simulink model "Zhang2004QP"  (Simulink 8.6)
settings: Solver=FixedStepAuto  StartTime=0.0  StopTime=20  FixedStep=Ts  RelTol=1e-3
InitFcn:
  | Zhang2004QP_init;
undefined symbols (not defined in the file or in its folder): CONFIG, DiscIntNeverNeededParam, model, ROBOT_DOF, Ts
libraries: WBToolboxLibrary x14
settings Model: Creator=marie  LastModifiedBy=marie
settings DataIOCC: SaveFormat=Dataset  SignalLoggingSaveFormat=Dataset
settings OptimizationCC: ExpressionDepthLimit=128
settings DebuggingCC: UnderspecifiedInitializationDetection=Simplified  MergeDetectMultiDrivingBlocksExec=error  SolverPrmCheckMsg=none  FcnCallInpInsideContextMsg=EnableAllAsError  StateNameClashWarn=none
settings HardwareCC: ProdBitPerPointer=64  ProdLargestAtomicFloat=Float  ProdIntDivRoundTo=Zero  ProdEndianess=LittleEndian  ProdWordSize=64  ProdHWDeviceType=Intel->x86-64 (Windows64)
settings GRTTargetCC: GeneratePreprocessorConditionals=Use local settings  CombineOutputUpdateFcns=on  GRTInterface=off
settings ConfigComp: CovModelRefEnable=off

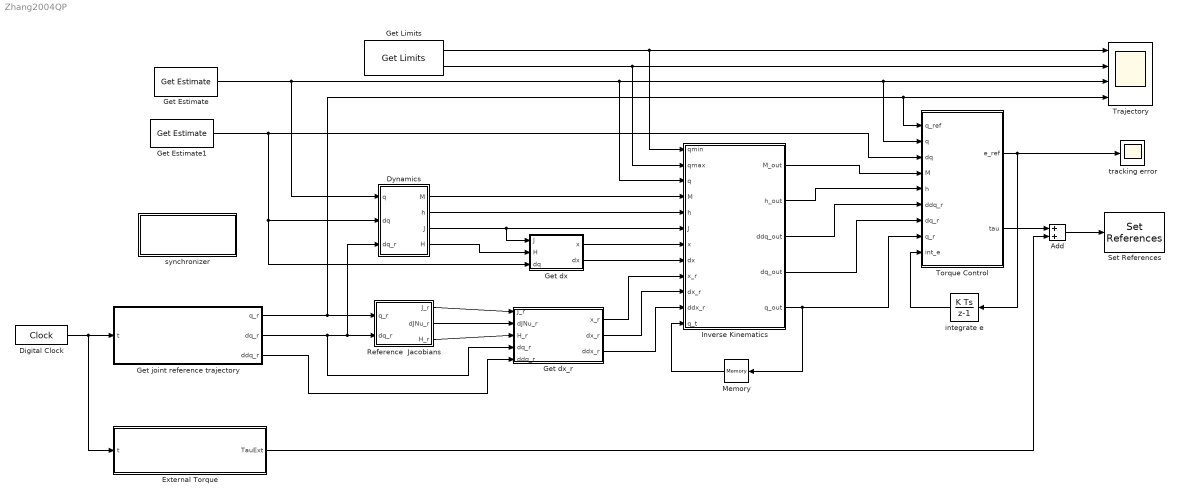
== system Zhang2004QP ==
  Add : Sum
  Digital Clock : DigitalClock  SampleTime=Ts
  Dynamics : Subsystem
  External Torque : MATLAB Function  TreatAsAtomicUnit=on
  Get Estimate : WBToolboxLibrary/wholeBodyStates/Get Estimate  estimateType=Joints Position  robotName=WBT_robotName  localName=WBT_modelName  wbiFile=WBT_wbiFilename  wbiList=WBT_wbiList
  Get Estimate1 : WBToolboxLibrary/wholeBodyStates/Get Estimate  estimateType=Joints Velocity  robotName=WBT_robotName  localName=WBT_modelName  wbiFile=WBT_wbiFilename  wbiList=WBT_wbiList
  Get Limits : WBToolboxLibrary/wholeBodyStates/Get Limits  limitsType=Position  robotName=WBT_robotName  localName=WBT_modelName  wbiFile=WBT_wbiFilename  wbiList=WBT_wbiList
  Get dx : MATLAB Function  TreatAsAtomicUnit=on
  Get dx_r : MATLAB Function  TreatAsAtomicUnit=on
  Get joint reference trajectory : MATLAB Function  TreatAsAtomicUnit=on
  Inverse Kinematics : MATLAB Function  TreatAsAtomicUnit=on
  Memory : Memory  InheritSampleTime=on
  Reference  Jacobians : Subsystem
  Set References : WBToolboxLibrary/wholeBodyActuators/Set References  controlType=Torque  robotName=WBT_robotName  localName=WBT_modelName  wbiFile=WBT_wbiFilename  wbiList=WBT_wbiList
  Torque Control : MATLAB Function  TreatAsAtomicUnit=on
  Trajectory : Scope  NumInputPorts=4
  integrate e : DiscreteIntegrator  InitialConditionSetting=State (most efficient)  SampleTime=Ts  ICPrevOutput=DiscIntNeverNeededParam  ICPrevScaledInput=DiscIntNeverNeededParam
  synchronizer : Subsystem
      mask Display: disp('SYNCHRONIZER')
  tracking error : Scope
  wires:
  Digital Clock/1 -> External Torque/1(t), Get joint reference trajectory/1(t)
  Torque Control/1(e_ref) -> integrate e/1, tracking error/1
  integrate e/1 -> Torque Control/9(int_e)
  Get Estimate/1 -> Dynamics/1(q), Trajectory/3, Torque Control/2(q), Inverse Kinematics/3(q)
  Get Estimate1/1 -> Get dx/3(dq), Dynamics/2(dq), Torque Control/3(dq)
  Get joint reference trajectory/1(q_r) -> Reference  Jacobians/1(q_r), Trajectory/4, Torque Control/1(q_ref)
  Get joint reference trajectory/2(dq_r) -> Reference  Jacobians/2(dq_r), Dynamics/3(dq_r), Get dx_r/4(dq_r)
  Get joint reference trajectory/3(ddq_r) -> Get dx_r/5(ddq_r)
  Get Limits/1 -> Trajectory/1, Inverse Kinematics/1(qmin)
  Get Limits/2 -> Trajectory/2, Inverse Kinematics/2(qmax)
  Dynamics/1(M) -> Inverse Kinematics/4(M)
  Dynamics/2(h) -> Inverse Kinematics/5(h)
  Reference  Jacobians/1(J_r) -> Get dx_r/1(J_r)
  Reference  Jacobians/2(dJNu_r) -> Get dx_r/2(dJNu_r)
  Dynamics/3(J) -> Inverse Kinematics/6(J), Get dx/1(J)
  Reference  Jacobians/3(H_r) -> Get dx_r/3(H_r)
  Dynamics/4(H) -> Get dx/2(H)
  Get dx_r/1(x_r) -> Inverse Kinematics/9(x_r)
  Get dx_r/2(dx_r) -> Inverse Kinematics/10(dx_r)
  Get dx_r/3(ddx_r) -> Inverse Kinematics/11(ddx_r)
  Get dx/1(x) -> Inverse Kinematics/7(x)
  Get dx/2(dx) -> Inverse Kinematics/8(dx)
  Inverse Kinematics/3(ddq_out) -> Torque Control/6(ddq_r)
  Inverse Kinematics/5(q_out) -> Torque Control/8(q_r), Memory/1
  Memory/1 -> Inverse Kinematics/12(q_t)
  Inverse Kinematics/1(M_out) -> Torque Control/4(M)
  Inverse Kinematics/2(h_out) -> Torque Control/5(h)
  Inverse Kinematics/4(dq_out) -> Torque Control/7(dq_r)
  Torque Control/2(tau) -> Add/1
  External Torque/1(TauExt) -> Add/2
  Add/1 -> Set References/1

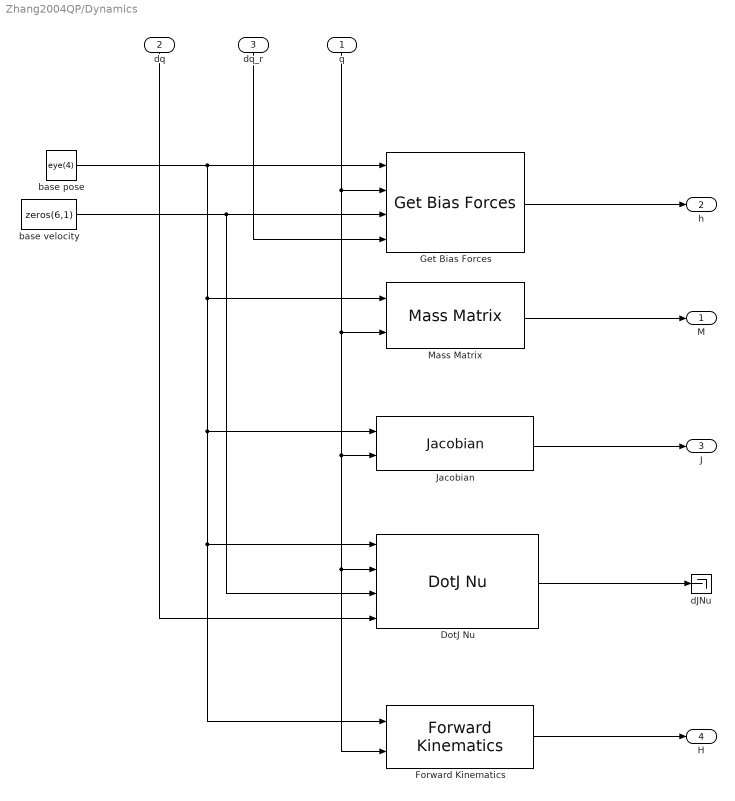
== system Zhang2004QP/Dynamics ==
  q : Inport
  dq : Inport  Port=2
  dq_r : Inport  Port=3
  DotJ Nu : WBToolboxLibrary/wholeBodyModel/Jacobians/DotJ Nu  frameName='r_sole'  robotName=WBT_robotName  localName=WBT_modelName  wbiFile=WBT_wbiFilename  wbiList=WBT_wbiList
  Forward Kinematics : WBToolboxLibrary/wholeBodyModel/Kinematics/Forward Kinematics  frameName='r_sole'  robotName=WBT_robotName  localName=WBT_modelName  wbiFile=WBT_wbiFilename  wbiList=WBT_wbiList
  Get Bias Forces : WBToolboxLibrary/wholeBodyModel/Dynamics/Get Bias Forces  robotName=WBT_robotName  localName=WBT_modelName  wbiFile=WBT_wbiFilename  wbiList=WBT_wbiList
  Jacobian : WBToolboxLibrary/wholeBodyModel/Jacobians/Jacobian  frameName='r_sole'  robotName=WBT_robotName  localName=WBT_modelName  wbiFile=WBT_wbiFilename  wbiList=WBT_wbiList
  Mass Matrix : WBToolboxLibrary/wholeBodyModel/Dynamics/Mass Matrix  robotName=WBT_robotName  localName=WBT_modelName  wbiFile=WBT_wbiFilename  wbiList=WBT_wbiList
  base pose : Constant  Value=eye(4)
  base velocity : Constant  Value=zeros(6,1)
  dJNu : Terminator
  M : Outport
  h : Outport  Port=2
  J : Outport  Port=3
  H : Outport  Port=4
  wires:
  base pose/1 -> Get Bias Forces/1, Forward Kinematics/1, DotJ Nu/1, Jacobian/1, Mass Matrix/1
  dq_r/1 -> Get Bias Forces/4
  Mass Matrix/1 -> M/1
  base velocity/1 -> DotJ Nu/3, Get Bias Forces/3
  Get Bias Forces/1 -> h/1
  q/1 -> DotJ Nu/2, Forward Kinematics/2, Jacobian/2, Mass Matrix/2, Get Bias Forces/2
  dq/1 -> DotJ Nu/4
  Jacobian/1 -> J/1
  DotJ Nu/1 -> dJNu/1
  Forward Kinematics/1 -> H/1

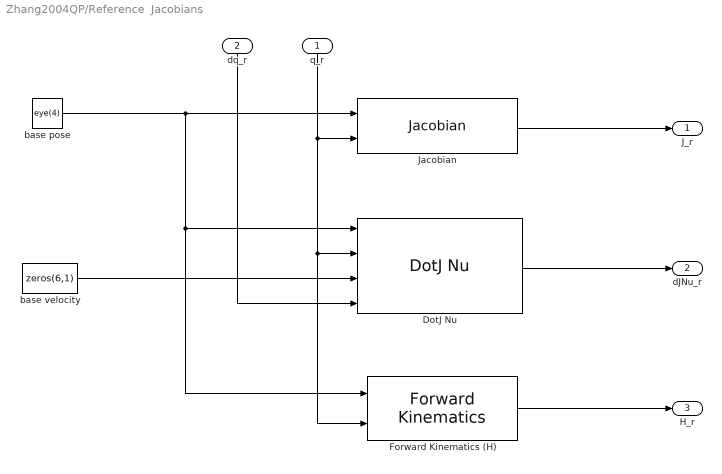
== system Zhang2004QP/Reference  Jacobians ==
  q_r : Inport
  dq_r : Inport  Port=2
  DotJ Nu : WBToolboxLibrary/wholeBodyModel/Jacobians/DotJ Nu  frameName='r_sole'  robotName=WBT_robotName  localName=WBT_modelName  wbiFile=WBT_wbiFilename  wbiList=WBT_wbiList
  Forward Kinematics (H) : WBToolboxLibrary/wholeBodyModel/Kinematics/Forward Kinematics  frameName='r_sole'  robotName=WBT_robotName  localName=WBT_modelName  wbiFile=WBT_wbiFilename  wbiList=WBT_wbiList
  Jacobian : WBToolboxLibrary/wholeBodyModel/Jacobians/Jacobian  frameName='r_sole'  robotName=WBT_robotName  localName=WBT_modelName  wbiFile=WBT_wbiFilename  wbiList=WBT_wbiList
  base pose : Constant  Value=eye(4)
  base velocity : Constant  Value=zeros(6,1)
  J_r : Outport
  dJNu_r : Outport  Port=2
  H_r : Outport  Port=3
  wires:
  DotJ Nu/1 -> dJNu_r/1
  Jacobian/1 -> J_r/1
  q_r/1 -> Jacobian/2, DotJ Nu/2, Forward Kinematics (H)/2
  base velocity/1 -> DotJ Nu/3
  base pose/1 -> Jacobian/1, Forward Kinematics (H)/1, DotJ Nu/1
  dq_r/1 -> DotJ Nu/4
  Forward Kinematics (H)/1 -> H_r/1

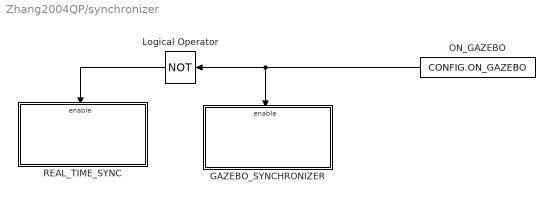
== system Zhang2004QP/synchronizer ==
  GAZEBO_SYNCHRONIZER : Subsystem
  Logical Operator : Logic  Operator=NOT  AllPortsSameDT=off  OutDataTypeStr=boolean
  "ON_GAZEBO " : Constant  Value=CONFIG.ON_GAZEBO
  REAL_TIME_SYNC : Subsystem
  wires:
  Logical Operator/1 -> REAL_TIME_SYNC/Enable
  "ON_GAZEBO "/1 -> GAZEBO_SYNCHRONIZER/Enable, Logical Operator/1

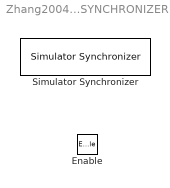
== system Zhang2004QP/synchronizer/GAZEBO_SYNCHRONIZER ==
  Enable : EnablePort
  Simulator Synchronizer : WBToolboxLibrary/Utilities/Simulator Synchronizer  period=CONFIG.Ts  serverPortName='/clock/rpc'  clientPortName='/WBT_synchronizer/rpc:o'

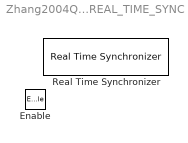
== system Zhang2004QP/synchronizer/REAL_TIME_SYNC ==
  Enable : EnablePort
  Real Time Synchronizer : WBToolboxLibrary/Utilities/Real Time Synchronizer  period=CONFIG.Ts

== matlab function Torque Control ==
  data: e_ref output double; q_ref input double; q input double; dq input double; M input double; h input double; ddq_r input double; dq_r input double; q_r input double; tau output double; int_e input double; ROBOT_DOF parameter double; model parameter double
function [e_ref, tau] = jointEvolutionControlFCN(q_ref, q, dq, M, h, ddq_r, dq_r, q_r, int_e, ROBOT_DOF, model)


[tau, e_ref] = jointEvolutionControl(q_ref, q, dq, M, h, ddq_r, dq_r, q_r, int_e, ROBOT_DOF, model);

== matlab function Get joint reference trajectory ==
  data: q_r output double; dq_r output double; ddq_r output double; t input double; model parameter double
function [q_r, dq_r, ddq_r] = generateReferenceTrajectoriesFCN(t, model)

[q_r, dq_r, ddq_r]  = generateReferenceTrajectories(t, model);

== matlab function Get dx_r ==
  data: x_r output double; J_r input double; dx_r output double; dJNu_r input double; H_r input double; dq_r input double; ddq_r input double; ddx_r output double
function [x_r, dx_r, ddx_r] = get_dx_rFCN(J_r, dJNu_r, H_r, dq_r, ddq_r)

%base velocity and acceleration = 0
Nu_r = [zeros(6,1); dq_r];
dNu_r = [zeros(6,1); ddq_r];

[x_r, dx_r, ddx_r] = get_dx(J_r, dJNu_r, H_r, Nu_r, dNu_r);

end

== matlab function Inverse Kinematics ==
  data: qmin input double; qmax input double; q input double; M input double; h input double; J input double; x input double; dx input double; x_r input double; M_out output double; h_out output double; ddq_out output double; dq_out output double; q_out output double; dx_r input double; ddx_r input double; q_t input double; Ts parameter double; ROBOT_DOF parameter double; model parameter double
function [M_out, h_out, ddq_out, dq_out, q_out] = qpInverseKinematicsFCN(qmin, qmax, q, M, h, J, x, dx, x_r, dx_r, ddx_r, q_t, Ts, ROBOT_DOF, model)


[ddq_out, dq_out, q_out] = qpInverseKinematics(qmin, qmax, q, M, h, J, x, dx, x_r, dx_r, ddx_r, q_t, Ts, ROBOT_DOF, model);


%Variables passing through
M_out = M;
h_out = h;

== matlab function External Torque ==
  data: TauExt output double; t input double; model parameter double
function TauExt = applyExternTorqueFCN(t, model)

TauExt = applyExternTorque(t, model);

== matlab function Get dx ==
  data: x output double; J input double; dx output double; H input double; dq input double
function [x, dx] = fcn(J, H, dq) %ddq, dJNu

%base velocity = 0
Nu = [zeros(6,1); dq];

[x, dx, ~] = get_dx(J, [], H, Nu, []);

end
